simulink model "rmxplorer_example1"  (R2019b)
settings: Solver=FixedStepAuto  StartTime=0.0  StopTime=inf  RelTol=1e-3  EnableMultiTasking=on
libraries: mbedblockslib x17, simulink x4
settings Model: SimulationMode=accelerator  SILPILModeSetting=veronly  ExtModeTrigDuration=10  Creator=pokpong.c  LastModifiedBy=szgno
settings SolverCC: PositivePriorityOrder=on
settings OptimizationCC: StrengthReduction=on  PassReuseOutputArgsAs=Individual arguments  ZeroExternalMemoryAtStartup=off  ZeroInternalMemoryAtStartup=off  MaxStackSize=64  OptimizeBlockOrder=speed  OptimizationPriority=Speed  OptimizationCustomize=off  MultiThreadedLoops=on  EfficientTunableParamExpr=on
settings DebuggingCC: ParameterTunabilityLossMsg=error
settings HardwareCC: ProdBitPerPointer=32  ProdBitPerSizeT=32  ProdBitPerPtrDiffT=32  ProdLargestAtomicInteger=Long  ProdLargestAtomicFloat=Double  ProdWordSize=32  ProdHWDeviceType=ARM Compatible->ARM Cortex
settings ModelReferenceCC: ModelReferenceNumInstancesAllowed=Single
settings SFSimCC: MATLABDynamicMemAlloc=off
settings RTWCC: SystemTargetFile=ert.tlc  HardwareBoard=STM32 Nucleo F411RE  TLCOptions=-aInlineSetEventsForThisBaseRateFcn=TLC_FALSE -aSuppressMultiTaskScheduler=TLC_FALSE -aRateBasedStepFcn=1  TemplateMakefile=ert_default_tmf  GenerateReport=on  Toolchain=GNU Tools for ARM Embedded Processors  IncludeHyperlinkInReport=on  LaunchReport=on  GenerateTraceInfo=on  GenerateTraceReport=on  GenerateTraceReportSl=on  GenerateTraceReportSf=on  GenerateTraceReportEml=on
settings CodeAppCC: ForceParamTrailComments=on  IgnoreCustomStorageClasses=off  OperatorAnnotations=on  SimulinkDataObjDesc=on  SFDataObjDesc=on  InsertBlockDesc=on
settings ERTTargetCC: SupportContinuousTime=on  ExtModeStaticAllocSize=2000

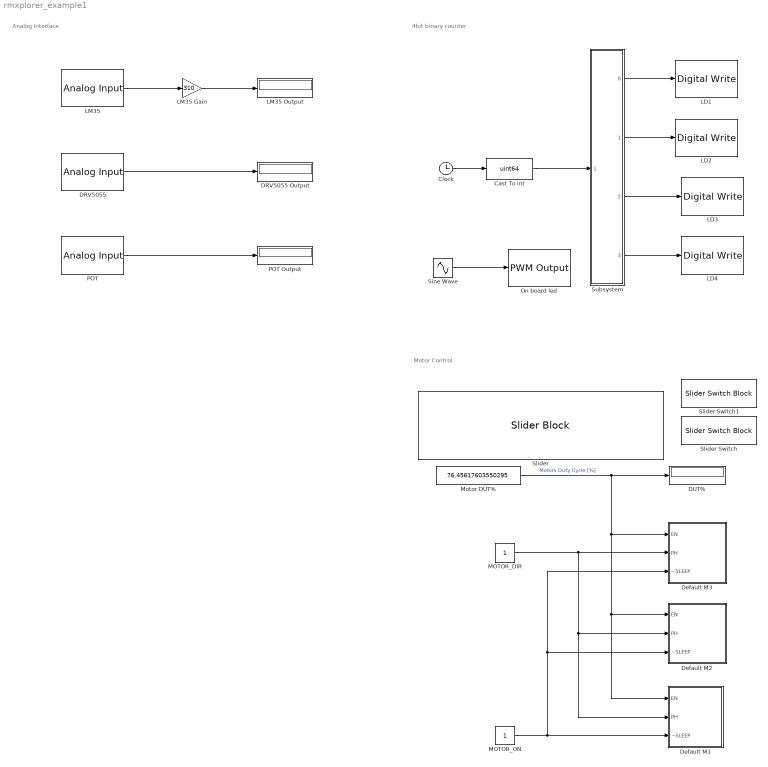
== system rmxplorer_example1 ==
  note: 4bit binary counter
  note: Motor Control
  note: Analog Interface
  Cast To int : DataTypeConversion  OutDataTypeStr=uint64
  Clock : Clock
  DRV5055 : mbedblockslib/Analog Input  Pin=PA_1  ReadResultsOnly=off  ConversionTriggerSource=Software  ExternalTriggerType=uint32( 0 )  OutputDataType=double  EnableConversionCompleteNotify=off  EnableOuputStatus=off  SampleTime=0.05
      settings: SourceProductName=Simulink Coder Support Package for BBC microbit Board  SourceProductBaseCode=MICROBIT
  DRV5055 Output : Display
  DUT% : Display
  Default M1 : Subsystem
  Default M2 : Subsystem
  Default M3 : Subsystem
  LD1 : mbedblockslib/Digital Write  Pin=PB_14  Direction=output
      settings: SourceProductName=Simulink Coder Support Package for BBC microbit Board  SourceProductBaseCode=MICROBIT
  LD2 : mbedblockslib/Digital Write  Pin=PA_13  Direction=output
      settings: SourceProductName=Simulink Coder Support Package for BBC microbit Board  SourceProductBaseCode=MICROBIT
  LD3 : mbedblockslib/Digital Write  Pin=PA_14  Direction=output
      settings: SourceProductName=Simulink Coder Support Package for BBC microbit Board  SourceProductBaseCode=MICROBIT
  LD4 : mbedblockslib/Digital Write  Pin=PC_13  Direction=output
      settings: SourceProductName=Simulink Coder Support Package for BBC microbit Board  SourceProductBaseCode=MICROBIT
  LM35 : mbedblockslib/Analog Input  Pin=PA_0  ReadResultsOnly=off  ConversionTriggerSource=Software  ExternalTriggerType=uint32( 0 )  OutputDataType=double  EnableConversionCompleteNotify=off  EnableOuputStatus=off  SampleTime=0.05
      settings: SourceProductName=Simulink Coder Support Package for BBC microbit Board  SourceProductBaseCode=MICROBIT
  LM35 Gain : Gain  Gain=310
  LM35 Output : Display
  MOTOR_DIR : Constant
  MOTOR_ON : Constant
  Motor DUT% : Constant  Value=76.45617603550295
  On board led : mbedblockslib/PWM Output  Pin=13  EnableInputFrequency=off  InitialFrequency=1000  InitialDutyCycle=0  NotificationType=None
      settings: SourceProductName=Simulink Coder Support Package for BBC microbit Board  SourceProductBaseCode=MICROBIT
  POT : mbedblockslib/Analog Input  Pin=PA_7  ReadResultsOnly=off  ConversionTriggerSource=Software  ExternalTriggerType=uint32( 0 )  OutputDataType=double  EnableConversionCompleteNotify=off  EnableOuputStatus=off  SampleTime=0.05
      settings: SourceProductName=Simulink Coder Support Package for BBC microbit Board  SourceProductBaseCode=MICROBIT
  POT Output : Display
  "Sine Wave " : Sin  Amplitude=50  Bias=50  Frequency=2  SampleTime=0
  Slider : SliderBlock
  Slider Switch : SliderSwitchBlock
      settings: Values={{'Off', 'On'}, [0 1]}
  Slider Switch1 : SliderSwitchBlock
      settings: Values={{'CW', 'CCW'}, [0 1]}
  Subsystem : Subsystem
  wires:
  LM35/1 -> LM35 Gain/1
  DRV5055/1 -> DRV5055 Output/1
  LM35 Gain/1 -> LM35 Output/1
  POT/1 -> POT Output/1
  "Sine Wave "/1 -> On board led/1
  Clock/1 -> Cast To int/1
  Cast To int/1 -> Subsystem/1(4 bit in)
  Subsystem/1(0) -> LD1/1
  Subsystem/2(1) -> LD2/1
  Subsystem/3(2) -> LD3/1
  Subsystem/4(3) -> LD4/1
  MOTOR_DIR/1 -> Default M3/2(PH), Default M1/2(PH), Default M2/2(PH)
  MOTOR_ON/1 -> Default M3/3(~SLEEP), Default M2/3(~SLEEP), Default M1/3(~SLEEP)
  Motor DUT%/1 -> Default M3/1(EN), Default M1/1(EN), Default M2/1(EN), DUT%/1  "Motors Duty Cycle [%]"

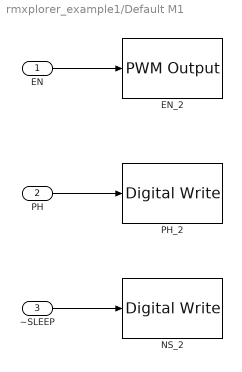
== system rmxplorer_example1/Default M1 ==
  EN : Inport
  PH : Inport  Port=2
  ~SLEEP : Inport  Port=3
  EN_2 : mbedblockslib/PWM Output  Pin=PA_11  EnableInputFrequency=off  InitialFrequency=300  InitialDutyCycle=50  NotificationType=None
      settings: SourceProductName=Simulink Coder Support Package for BBC microbit Board  SourceProductBaseCode=MICROBIT
  NS_2 : mbedblockslib/Digital Write  Pin=PB_2  Direction=output
      settings: SourceProductName=Simulink Coder Support Package for BBC microbit Board  SourceProductBaseCode=MICROBIT
  PH_2 : mbedblockslib/Digital Write  Pin=PC_7  Direction=output
      settings: SourceProductName=Simulink Coder Support Package for BBC microbit Board  SourceProductBaseCode=MICROBIT
  wires:
  ~SLEEP/1 -> NS_2/1
  EN/1 -> EN_2/1
  PH/1 -> PH_2/1

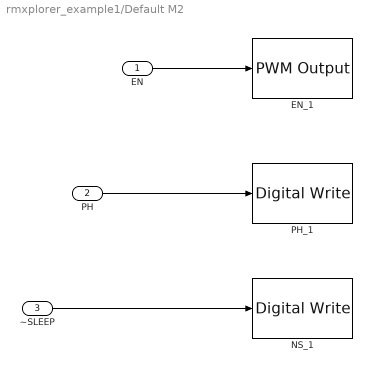
== system rmxplorer_example1/Default M2 ==
  EN : Inport
  PH : Inport  Port=2
  ~SLEEP : Inport  Port=3
  EN_1 : mbedblockslib/PWM Output  Pin=PC_8  EnableInputFrequency=off  InitialFrequency=300  InitialDutyCycle=50  NotificationType=None
      settings: SourceProductName=Simulink Coder Support Package for BBC microbit Board  SourceProductBaseCode=MICROBIT
  NS_1 : mbedblockslib/Digital Write  Pin=PA_12  Direction=output
      settings: SourceProductName=Simulink Coder Support Package for BBC microbit Board  SourceProductBaseCode=MICROBIT
  PH_1 : mbedblockslib/Digital Write  Pin=PC_6  Direction=output
      settings: SourceProductName=Simulink Coder Support Package for BBC microbit Board  SourceProductBaseCode=MICROBIT
  wires:
  PH/1 -> PH_1/1
  ~SLEEP/1 -> NS_1/1
  EN/1 -> EN_1/1

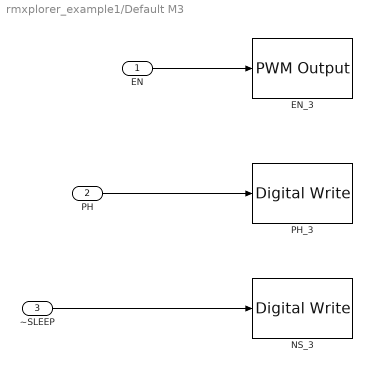
== system rmxplorer_example1/Default M3 ==
  EN : Inport
  PH : Inport  Port=2
  ~SLEEP : Inport  Port=3
  EN_3 : mbedblockslib/PWM Output  Pin=PA_9  EnableInputFrequency=off  InitialFrequency=300  InitialDutyCycle=50  NotificationType=None
      settings: SourceProductName=Simulink Coder Support Package for BBC microbit Board  SourceProductBaseCode=MICROBIT
  NS_3 : mbedblockslib/Digital Write  Pin=PB_15  Direction=output
      settings: SourceProductName=Simulink Coder Support Package for BBC microbit Board  SourceProductBaseCode=MICROBIT
  PH_3 : mbedblockslib/Digital Write  Pin=PB_10  Direction=output
      settings: SourceProductName=Simulink Coder Support Package for BBC microbit Board  SourceProductBaseCode=MICROBIT
  wires:
  PH/1 -> PH_3/1
  ~SLEEP/1 -> NS_3/1
  EN/1 -> EN_3/1

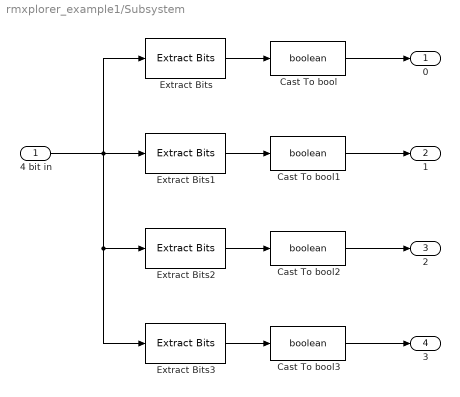
== system rmxplorer_example1/Subsystem ==
  4 bit in : Inport
  Cast To bool{,1..3} (4 alike) : DataTypeConversion  OutDataTypeStr=boolean
  Extract Bits : simulink/Logic and Bit Operations/Extract Bits  bitsToExtract=Range of bits  numBits=8  bitIdxRange=0  outScalingMode=Treat bit field as an integer
      settings: SourceProductName=Simulink
  Extract Bits1 : simulink/Logic and Bit Operations/Extract Bits  bitsToExtract=Range of bits  numBits=8  bitIdxRange=1  outScalingMode=Treat bit field as an integer
      settings: SourceProductName=Simulink
  Extract Bits2 : simulink/Logic and Bit Operations/Extract Bits  bitsToExtract=Range of bits  numBits=8  bitIdxRange=2  outScalingMode=Treat bit field as an integer
      settings: SourceProductName=Simulink
  Extract Bits3 : simulink/Logic and Bit Operations/Extract Bits  bitsToExtract=Range of bits  numBits=8  bitIdxRange=3  outScalingMode=Treat bit field as an integer
      settings: SourceProductName=Simulink
  0 : Outport
  1 : Outport  Port=2
  2 : Outport  Port=3
  3 : Outport  Port=4
  wires:
  Extract Bits1/1 -> Cast To bool1/1
  4 bit in/1 -> Extract Bits3/1, Extract Bits2/1, Extract Bits1/1, Extract Bits/1
  Extract Bits/1 -> Cast To bool/1
  Cast To bool3/1 -> 3/1
  Extract Bits3/1 -> Cast To bool3/1
  Cast To bool/1 -> 0/1
  Extract Bits2/1 -> Cast To bool2/1
  Cast To bool1/1 -> 1/1
  Cast To bool2/1 -> 2/1
